simulink model "verify_Flow_Diverter_mdl"  (R2016b)
settings: Solver=ode45  StartTime=0.0  StopTime=75  MaxStep=1  RelTol=1e-3  EnableMultiTasking=on
libraries: carnot x2, simulink x1
settings Model: Creator=drhf  LastModifiedBy=drhf
settings DataIOCC: SaveFormat=Array  SignalLoggingSaveFormat=ModelDataLogs
settings OptimizationCC: ExpressionDepthLimit=2147483647  LifeSpan=inf
settings DebuggingCC: UnderspecifiedInitializationDetection=Classic  MergeDetectMultiDrivingBlocksExec=none  SolverPrmCheckMsg=warning  FcnCallInpInsideContextMsg=warning  StateNameClashWarn=warning  SFUnexpectedBacktrackingDiag=warning  SFNoUnconditionalDefaultTransitionDiag=warning  SFExecutionAtInitializationDiag=none
settings HardwareCC: ProdBitPerPointer=32  ProdBitPerSizeT=32  ProdBitPerPtrDiffT=32  ProdLargestAtomicFloat=None  ProdIntDivRoundTo=Undefined  ProdEndianess=Unspecified  ProdWordSize=32  ProdHWDeviceType=32-bit Generic
settings ModelReferenceCC: PropagateSignalLabelsOutOfModel=off
settings GRTTargetCC: TargetLangStandard=C89/C90 (ANSI)  GeneratePreprocessorConditionals=Disable all  CombineOutputUpdateFcns=off  GRTInterface=on
settings ConfigComp: CovMetricSettings=dw  CovHtmlReporting=on  CovSaveCumulativeToWorkspaceVar=on  CovSaveSingleToWorkspaceVar=on  CovExternalEMLEnable=off

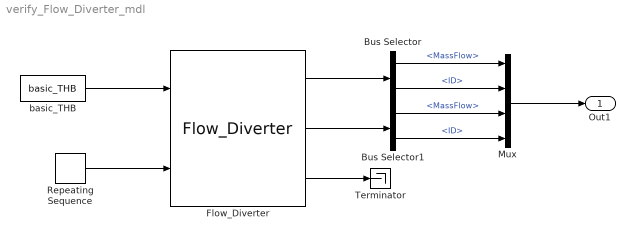
== system verify_Flow_Diverter_mdl ==
  Bus Selector : BusSelector  OutputSignals=MassFlow,ID
  Bus Selector1 : BusSelector  OutputSignals=MassFlow,ID
  Flow_Diverter : carnot/Hydraulics/Flow_Diverter
  Mux : Mux
  Repeating Sequence : simulink/Sources/Repeating Sequence  rep_seq_t=[0 20 60 80]  rep_seq_y=[1 1 0 0]
  Terminator : Terminator
  basic_THB : carnot/Basic/Hydraulics/basic_THB  t=20  mdot=600/3600  p=1e5  ID=No Pressure Drop  fluid=Water  mix=0  mix2=0  mix3=0  dia=0.02  hgt=0
  Out1 : Outport
  wires:
  Mux/1 -> Out1/1
  basic_THB/1 -> Flow_Diverter/1
  Repeating Sequence/1 -> Flow_Diverter/2
  Flow_Diverter/3 -> Terminator/1
  Flow_Diverter/1 -> Bus Selector/1
  Flow_Diverter/2 -> Bus Selector1/1
  Bus Selector/1 -> Mux/1  "<MassFlow>"
  Bus Selector/2 -> Mux/2  "<ID>"
  Bus Selector1/1 -> Mux/3  "<MassFlow>"
  Bus Selector1/2 -> Mux/4  "<ID>"
